simulink model "dc_model"  (R2025a)
settings: Solver=VariableStepAuto  StartTime=0.0  StopTime=5.0  RelTol=1e-3
undefined symbols (not defined in the file): b, J, K, L, R
settings Model: Creator=AN  LastModifiedBy=AN

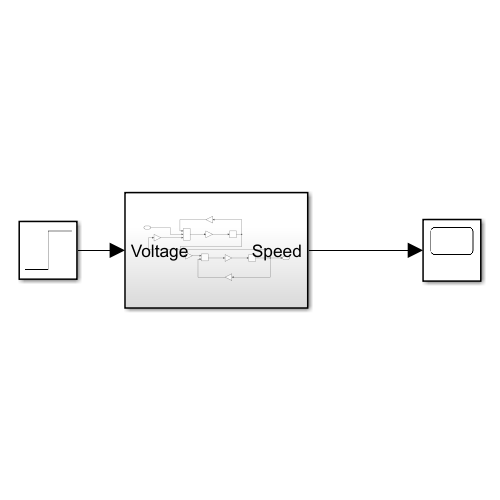
[thumbnail: Simulink's stored preview of the top-level diagram]
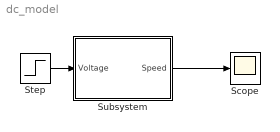
== system dc_model ==
  Scope : Scope
  Step : Step  Time=0  SampleTime=0
  Subsystem : Subsystem
  wires:
  Subsystem/1(Speed) -> Scope/1
  Step/1 -> Subsystem/1(Voltage)

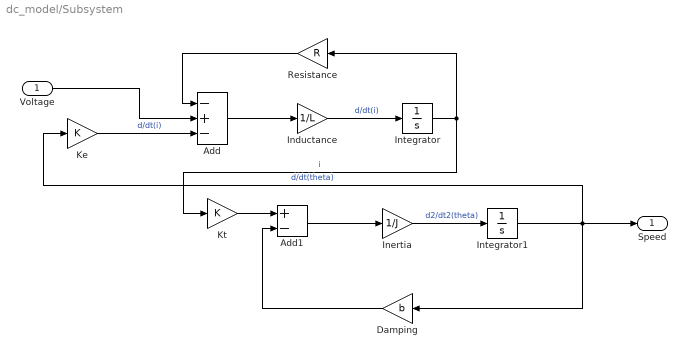
== system dc_model/Subsystem ==
  Voltage : Inport
  Add : Sum  Inputs=-+-
  Add1 : Sum  Inputs=+-
  Damping : Gain  Gain=b
  Inductance : Gain  Gain=1/L
  Inertia : Gain  Gain=1/J
  Integrator : Integrator
  Integrator1 : Integrator
  Ke : Gain  Gain=K
  Kt : Gain  Gain=K
  Resistance : Gain  Gain=R
  Speed : Outport
  wires:
  Kt/1 -> Add1/1
  Integrator/1 -> Resistance/1, Kt/1  "i"
  Integrator1/1 -> Speed/1, Ke/1, Damping/1  "d/dt(theta)"
  Add1/1 -> Inertia/1
  Ke/1 -> Add/3  "d/dt(i)"
  Inductance/1 -> Integrator/1  "d/dt(i)"
  Voltage/1 -> Add/2
  Add/1 -> Inductance/1
  Inertia/1 -> Integrator1/1  "d2/dt2(theta)"
  Resistance/1 -> Add/1
  Damping/1 -> Add1/2
